simulink model "przestrzen_stanu_1"  (R2014b)
settings: Solver=ode45  StartTime=0.0  StopTime=100.0  RelTol=1e-3
values from neighbouring files (symbols this model uses):
  A1 = [ - den_z(2:end); 1 0 0; 0 1 0 ]    [zad_2.m]
  C1 = [ num_z(2:end) ]    [zad_2.m]
undefined symbols (not defined in the file or in its folder): Tp, x0
settings Model: Creator=Konrad  LastModifiedBy=Konrad

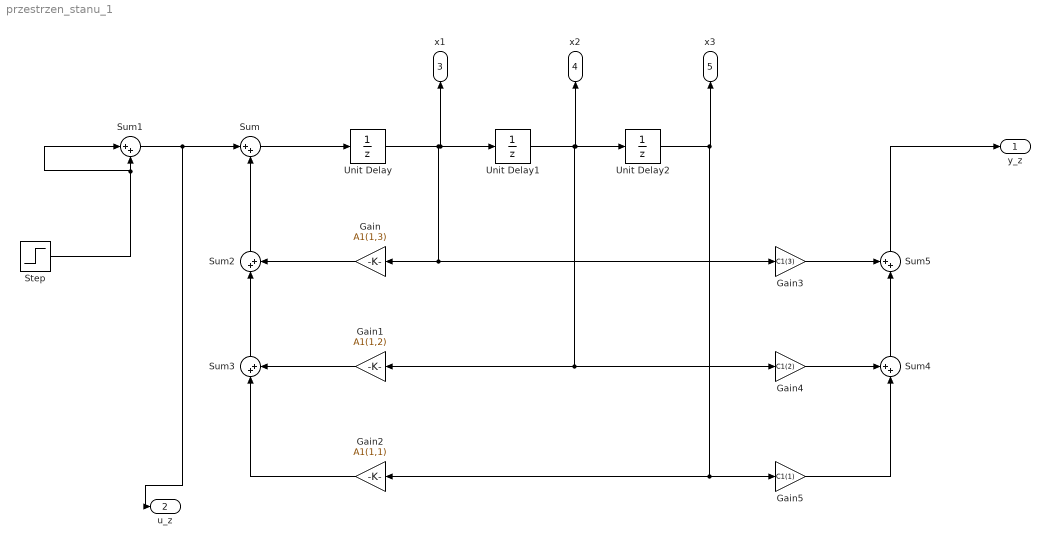
== system przestrzen_stanu_1 ==
  Gain : Gain  Gain=A1(1,3)
  Gain1 : Gain  Gain=A1(1,2)
  Gain2 : Gain  Gain=A1(1,1)
  Gain3 : Gain  Gain=C1(3)
  Gain4 : Gain  Gain=C1(2)
  Gain5 : Gain  Gain=C1(1)
  Step : Step  SampleTime=0
  Sum{,1..3} (4 alike) : Sum  Inputs=|++
  Sum4 : Sum  Inputs=++|
  Sum5 : Sum  Inputs=++|
  Unit Delay : UnitDelay  InitialCondition=x0(1)  SampleTime=Tp
  Unit Delay1 : UnitDelay  InitialCondition=x0(2)  SampleTime=Tp
  Unit Delay2 : UnitDelay  InitialCondition=x0(3)  SampleTime=Tp
  y_z : Outport
  u_z : Outport  Port=2
  x1 : Outport  Port=3
  x2 : Outport  Port=4
  x3 : Outport  Port=5
  wires:
  Unit Delay/1 -> Unit Delay1/1, x1/1, Gain3/1, Gain/1
  Unit Delay1/1 -> Unit Delay2/1, x2/1, Gain4/1, Gain1/1
  Sum/1 -> Unit Delay/1
  Sum2/1 -> Sum/2
  Sum3/1 -> Sum2/1
  Gain2/1 -> Sum3/1
  Unit Delay2/1 -> x3/1, Gain5/1, Gain2/1
  Gain1/1 -> Sum3/2
  Gain/1 -> Sum2/2
  Gain4/1 -> Sum4/1
  Gain3/1 -> Sum5/1
  Gain5/1 -> Sum4/2
  Sum4/1 -> Sum5/2
  Sum1/1 -> u_z/1, Sum/1
  Step/1 -> Sum1/1, Sum1/2
  Sum5/1 -> y_z/1
